simulink model "DCMotorModelVideoLecture"  (R2024b)
settings: Solver=VariableStepAuto  StartTime=0.0  StopTime=10.0  RelTol=1e-3
values from neighbouring files (symbols this model uses):
  B = [0 0 0 ... (first row only)    [satellitemodel2711.m]
undefined symbols (not defined in the file or in its folder): KePhi, Ra, tau_a, tau_m, TL, Va
settings Model: Creator=LEGION  LastModifiedBy=LEGION

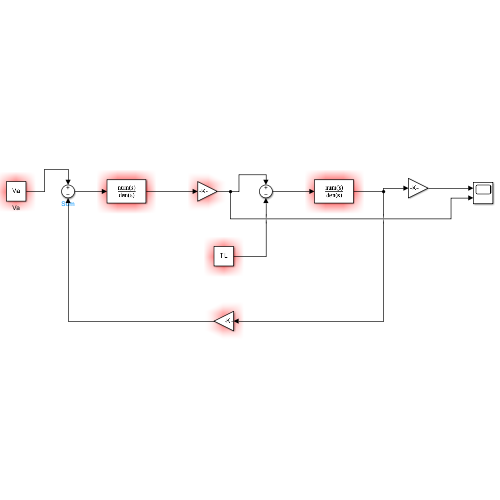
[thumbnail: Simulink's stored preview of the top-level diagram]
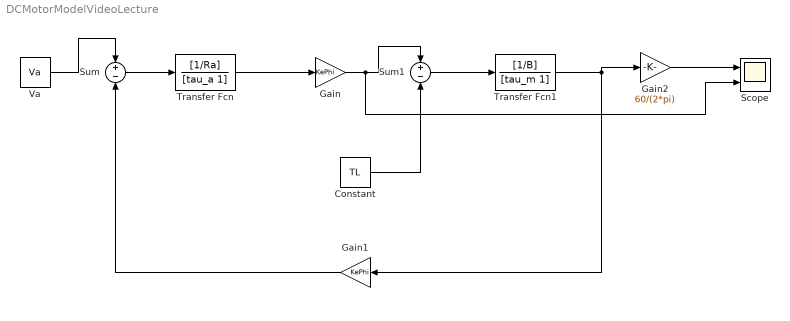
== system DCMotorModelVideoLecture ==
  Constant : Constant  Value=TL
  Gain : Gain  Gain=KePhi
  Gain1 : Gain  Gain=KePhi
  Gain2 : Gain  Gain=60/(2*pi)
  Scope : Scope  NumInputPorts=2
  Sum : Sum  Inputs=+-
  Sum1 : Sum  Inputs=+-
  Transfer Fcn : TransferFcn  Numerator=[1/Ra]  Denominator=[tau_a 1]
  Transfer Fcn1 : TransferFcn  Numerator=[1/B]  Denominator=[tau_m 1]
  Va : Constant  Value=Va
  wires:
  Va/1 -> Sum/1
  Sum/1 -> Transfer Fcn/1
  Transfer Fcn/1 -> Gain/1
  Gain/1 -> Scope/2, Sum1/1
  Constant/1 -> Sum1/2
  Sum1/1 -> Transfer Fcn1/1
  Transfer Fcn1/1 -> Gain1/1, Gain2/1
  Gain1/1 -> Sum/2
  Gain2/1 -> Scope/1
